simulink model "lab3_1"  (R2020a)
settings: Solver=VariableStepAuto  StartTime=0.0  StopTime=30.0  RelTol=1e-10  AbsTol=1e-10
values from neighbouring files (symbols this model uses):
  dbar = g*sin(theta)    [Lab3.m]
  vdes = 14    [Lab3.m]
libraries: cstblocks x2
settings Model: Creator=paulosga  LastModifiedBy=paulosga

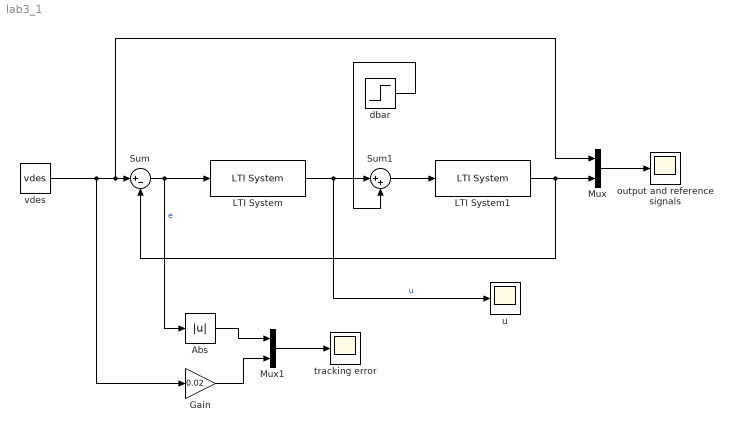
== system lab3_1 ==
  Abs : Abs
  Gain : Gain  Gain=0.02
  LTI System : cstblocks/LTI System  sys=C  IC=[]
  LTI System1 : cstblocks/LTI System  sys=G  IC=[]
  Mux : Mux  Inputs=2
  Mux1 : Mux  Inputs=2
  Sum : Sum  Inputs=|+-
  Sum1 : Sum  Inputs=|++
  dbar : Step  Time=15  After=dbar  SampleTime=0
  output and reference signals : Scope
  tracking error : Scope
  u : Scope
  vdes : Constant  Value=vdes
  wires:
  vdes/1 -> Gain/1, Mux/1, Sum/1
  Sum/1 -> LTI System/1, Abs/1  "e"
  LTI System/1 -> u/1, Sum1/1  "u"
  Sum1/1 -> LTI System1/1
  LTI System1/1 -> Mux/2, Sum/2
  Mux/1 -> output and reference signals/1
  dbar/1 -> Sum1/2
  Gain/1 -> Mux1/2
  Abs/1 -> Mux1/1
  Mux1/1 -> tracking error/1
